simulink model "week3problem3"  (R2020b)
settings: Solver=VariableStepAuto  StartTime=0.0  StopTime=10.0  RelTol=1e-3
values from neighbouring files (symbols this model uses):
  g = 9.81    [problem3.m]
  m = 1200    [problem3.m]
  R = 0.28    [problem3.m]
  V0 = 28    [problem3.m]
settings Model: Creator=Puru Gawande  LastModifiedBy=Puru Gawande

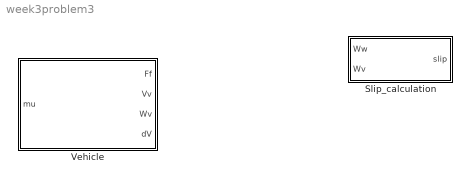
== system week3problem3 ==
  Slip_calculation : Subsystem
  Vehicle : Subsystem

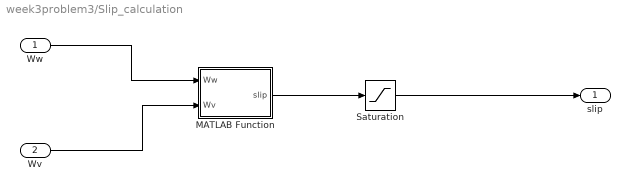
== system week3problem3/Slip_calculation ==
  Ww : Inport
  Wv : Inport  Port=2
  MATLAB Function : MATLAB Function  TreatAsAtomicUnit=on
  Saturation : Saturate  UpperLimit=1  LowerLimit=0
  slip : Outport
  wires:
  Ww/1 -> MATLAB Function/1(Ww)
  Wv/1 -> MATLAB Function/2(Wv)
  MATLAB Function/1(slip) -> Saturation/1
  Saturation/1 -> slip/1

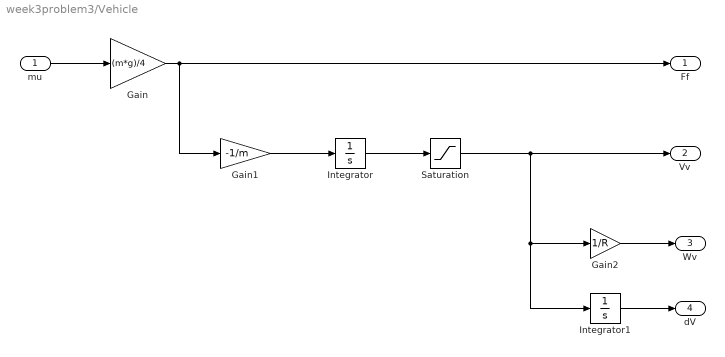
== system week3problem3/Vehicle ==
  mu : Inport
  Gain : Gain  Gain=(m*g)/4
  Gain1 : Gain  Gain=-1/m
  Gain2 : Gain  Gain=1/R
  Integrator : Integrator  InitialCondition=V0
  Integrator1 : Integrator
  Saturation : Saturate  UpperLimit=1000  LowerLimit=0.001
  Ff : Outport
  Vv : Outport  Port=2
  Wv : Outport  Port=3
  dV : Outport  Port=4
  wires:
  mu/1 -> Gain/1
  Gain/1 -> Gain1/1, Ff/1
  Gain1/1 -> Integrator/1
  Integrator/1 -> Saturation/1
  Saturation/1 -> Integrator1/1, Gain2/1, Vv/1
  Gain2/1 -> Wv/1
  Integrator1/1 -> dV/1

== matlab function week3problem3/Slip_calculation/MATLAB Function ==
  data: Ww input; slip output; Wv input
function slip = fcn(Ww, Wv)

slip=1-(Ww/(Wv+(Wv==0)*eps));
